simulink model "vehicle_lateral_model"  (Simulink 8.2)
settings: Solver=ode45  StartTime=0.0  StopTime=Tfinal  RelTol=1e-3
values from neighbouring files (symbols this model uses):
  Calpha = 39000    [vehicle_lateral_model_setup.m]
  Izz = 5428    [vehicle_lateral_model_setup.m]
  K = 19    [vehicle_lateral_model_setup.m]
  lf = 1.488    [vehicle_lateral_model_setup.m]
  lr = 1.712    [vehicle_lateral_model_setup.m]
  m = 2045    [vehicle_lateral_model_setup.m]
  mu = 0.9    [vehicle_lateral_model_setup.m]
  SteerAngle = 3*pi/180    (= 0.0523598775598)    [vehicle_lateral_model_setup.m]
  Vx_const = 80/3.6    (= 22.2222222222)    [vehicle_lateral_model_setup.m]
  Vy0 = 0    [vehicle_lateral_model_setup.m]
  X0 = 0    [vehicle_lateral_model_setup.m]
  Y0 = 0    [vehicle_lateral_model_setup.m]
  Yaw0 = 0    [vehicle_lateral_model_setup.m]
  yaw_rate0 = 0    [vehicle_lateral_model_setup.m]
settings Model: Creator=user  LastModifiedBy=edward
settings OptimizationCC: InitFltsAndDblsToZero=on

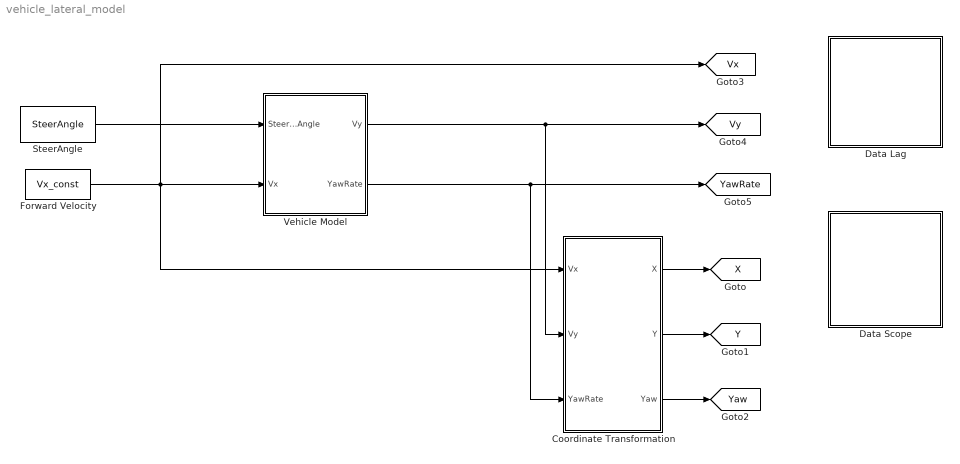
== system vehicle_lateral_model ==
  Coordinate Transformation : Subsystem
  Data Lag : Subsystem
  Data Scope : Subsystem
  Forward Velocity : Constant  Value=Vx_const
  SteerAngle : Constant  Value=SteerAngle
  Vehicle Model : Subsystem
  tag scope: Vx=global, Vy=global, X=global, Y=global, Yaw=global, YawRate=global
  wires:
  SteerAngle/1 -> Vehicle Model/1(Steering_Angle)
  Forward Velocity/1 -> Vehicle Model/2(Vx), [Vx], Coordinate Transformation/1(Vx)
  Vehicle Model/1(Vy) -> Coordinate Transformation/2(Vy), [Vy]
  Vehicle Model/2(YawRate) -> Coordinate Transformation/3(YawRate), [YawRate]
  Coordinate Transformation/1(X) -> [X]
  Coordinate Transformation/2(Y) -> [Y]
  Coordinate Transformation/3(Yaw) -> [Yaw]

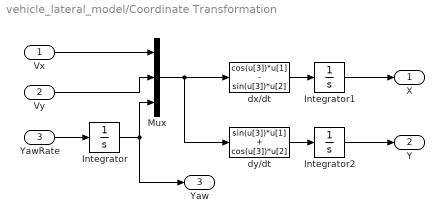
== system vehicle_lateral_model/Coordinate Transformation ==
  Vx : Inport
  Vy : Inport  Port=2
  YawRate : Inport  Port=3
  Integrator : Integrator  InitialCondition=Yaw0
  Integrator1 : Integrator  InitialCondition=X0
  Integrator2 : Integrator  InitialCondition=Y0
  Mux : Mux  Inputs=3
  dx/dt : Fcn  Expr=cos(u[3])*u[1] - sin(u[3])*u[2]
  dy/dt : Fcn  Expr=sin(u[3])*u[1] + cos(u[3])*u[2]
  X : Outport
  Y : Outport  Port=2
  Yaw : Outport  Port=3
  wires:
  YawRate/1 -> Integrator/1
  Vx/1 -> Mux/1
  Vy/1 -> Mux/2
  Integrator/1 -> Mux/3, Yaw/1
  Mux/1 -> dx/dt/1, dy/dt/1
  dx/dt/1 -> Integrator1/1
  Integrator1/1 -> X/1
  dy/dt/1 -> Integrator2/1
  Integrator2/1 -> Y/1

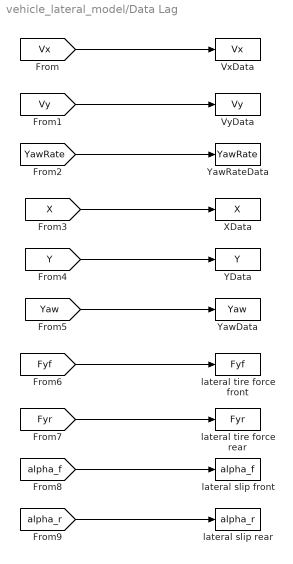
== system vehicle_lateral_model/Data Lag ==
  VxData : ToWorkspace  VariableName=Vx  SampleTime=-1
  VyData : ToWorkspace  VariableName=Vy  SampleTime=-1
  XData : ToWorkspace  VariableName=X  SampleTime=-1
  YData : ToWorkspace  VariableName=Y  SampleTime=-1
  YawData : ToWorkspace  VariableName=Yaw  SampleTime=-1
  YawRateData : ToWorkspace  VariableName=YawRate  SampleTime=-1
  lateral slip front : ToWorkspace  VariableName=alpha_f  SampleTime=-1
  lateral slip rear : ToWorkspace  VariableName=alpha_r  SampleTime=-1
  lateral tire force front : ToWorkspace  VariableName=Fyf  SampleTime=-1
  lateral tire force rear : ToWorkspace  VariableName=Fyr  SampleTime=-1
  wires:
  [Vx] -> VxData/1
  [Vy] -> VyData/1
  [YawRate] -> YawRateData/1
  [X] -> XData/1
  [Y] -> YData/1
  [Yaw] -> YawData/1
  [Fyf] -> lateral tire force front/1
  [Fyr] -> lateral tire force rear/1
  [alpha_f] -> lateral slip front/1
  [alpha_r] -> lateral slip rear/1

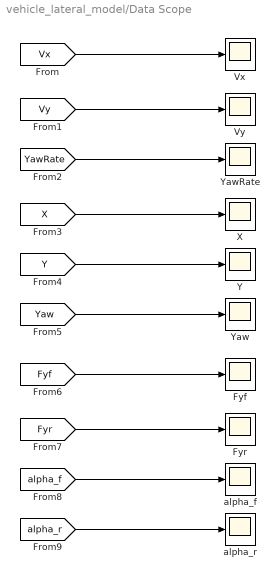
== system vehicle_lateral_model/Data Scope ==
  Fyf : Scope
  Fyr : Scope
      settings: SaveName=ScopeData3
  Vx : Scope
      settings: SaveName=ScopeData2
  Vy : Scope
      settings: SaveName=ScopeData4
  X : Scope
      settings: YMin=73.5393  YMax=81.2803  SaveName=ScopeData5
  Y : Scope
      settings: SaveName=ScopeData6
  Yaw : Scope
      settings: SaveName=ScopeData10
  YawRate : Scope
      settings: YMin=23.7489  YMax=26.2487  SaveName=ScopeData11
  alpha_f : Scope
      settings: YMin=23.7489  YMax=26.2487  SaveName=ScopeData8
  alpha_r : Scope
      settings: YMin=73.5393  YMax=81.2803  SaveName=ScopeData7
  wires:
  [Vx] -> Vx/1
  [Vy] -> Vy/1
  [YawRate] -> YawRate/1
  [X] -> X/1
  [Y] -> Y/1
  [Yaw] -> Yaw/1
  [Fyf] -> Fyf/1
  [Fyr] -> Fyr/1
  [alpha_f] -> alpha_f/1
  [alpha_r] -> alpha_r/1

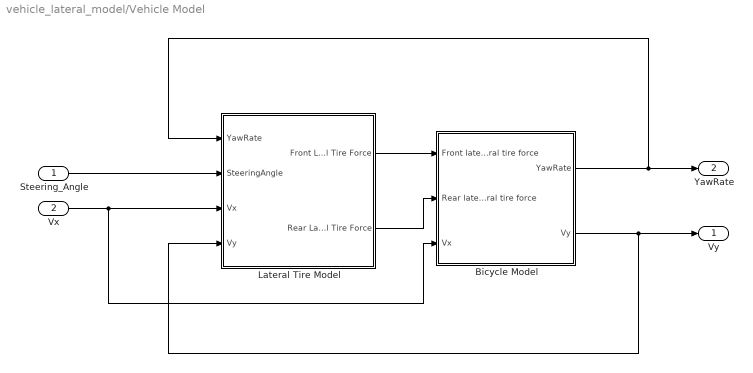
== system vehicle_lateral_model/Vehicle Model ==
  Steering_Angle : Inport
  Vx : Inport  Port=2
  Bicycle Model : Subsystem
  Lateral Tire Model : Subsystem
  Vy : Outport
  YawRate : Outport  Port=2
  wires:
  Steering_Angle/1 -> Lateral Tire Model/2(SteeringAngle)
  Lateral Tire Model/1(Front Lateral Tire Force) -> Bicycle Model/1(Front lateral tire force)
  Lateral Tire Model/2(Rear Lateral Tire Force) -> Bicycle Model/2(Rear lateral tire force)
  Bicycle Model/1(YawRate) -> Lateral Tire Model/1(YawRate), YawRate/1
  Bicycle Model/2(Vy) -> Vy/1, Lateral Tire Model/4(Vy)
  Vx/1 -> Lateral Tire Model/3(Vx), Bicycle Model/3(Vx)

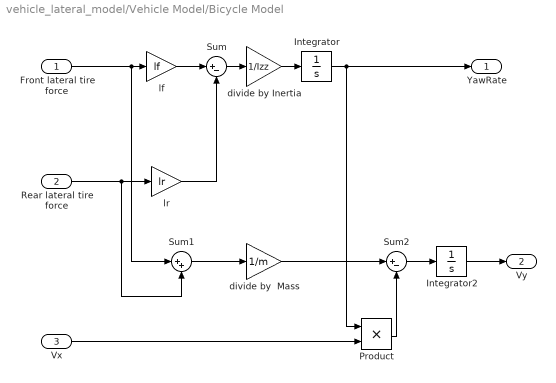
== system vehicle_lateral_model/Vehicle Model/Bicycle Model ==
  Front lateral tire force : Inport
  Rear lateral tire force : Inport  Port=2
  Vx : Inport  Port=3
  Integrator : Integrator  InitialCondition=yaw_rate0
  Integrator2 : Integrator  InitialCondition=Vy0
  Product : Product  RndMeth=Zero
  Sum : Sum  Inputs=|+-
  Sum1 : Sum  Inputs=|++
  Sum2 : Sum  Inputs=|+-
  divide by Inertia : Gain  Gain=1/Izz
  divide by  Mass : Gain  Gain=1/m
  lf : Gain  Gain=lf
  lr : Gain  Gain=lr
  YawRate : Outport
  Vy : Outport  Port=2
  wires:
  Front lateral tire force/1 -> lf/1, Sum1/1
  Rear lateral tire force/1 -> lr/1, Sum1/2
  lf/1 -> Sum/1
  lr/1 -> Sum/2
  Sum/1 -> divide by Inertia/1
  divide by Inertia/1 -> Integrator/1
  Integrator/1 -> YawRate/1, Product/1
  Sum1/1 -> divide by  Mass/1
  divide by  Mass/1 -> Sum2/1
  Vx/1 -> Product/2
  Product/1 -> Sum2/2
  Sum2/1 -> Integrator2/1
  Integrator2/1 -> Vy/1

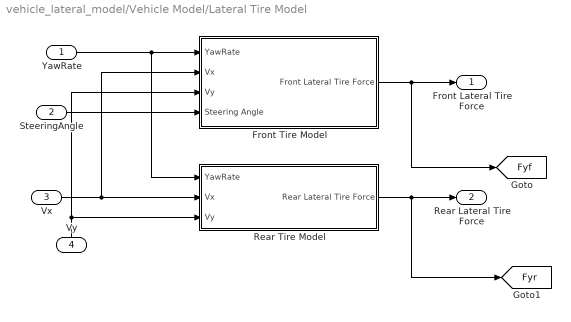
== system vehicle_lateral_model/Vehicle Model/Lateral Tire Model ==
  YawRate : Inport
  SteeringAngle : Inport  Port=2
  Vx : Inport  Port=3
  Vy : Inport  Port=4
  Front Tire Model : Subsystem
  Rear Tire Model : Subsystem
  Front Lateral Tire Force : Outport
  Rear Lateral Tire Force : Outport  Port=2
  tag scope: Fyf=global, Fyr=global
  wires:
  Vx/1 -> Rear Tire Model/2(Vx), Front Tire Model/2(Vx)
  Vy/1 -> Rear Tire Model/3(Vy), Front Tire Model/3(Vy)
  YawRate/1 -> Front Tire Model/1(YawRate), Rear Tire Model/1(YawRate)
  Front Tire Model/1(Front Lateral Tire Force) -> Front Lateral Tire Force/1, [Fyf]
  SteeringAngle/1 -> Front Tire Model/4(Steering Angle)
  Rear Tire Model/1(Rear Lateral Tire Force) -> Rear Lateral Tire Force/1, [Fyr]

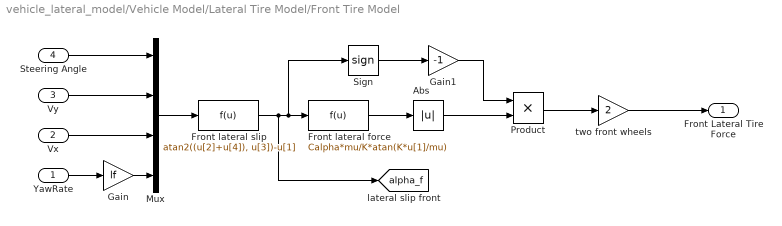
== system vehicle_lateral_model/Vehicle Model/Lateral Tire Model/Front Tire Model ==
  YawRate : Inport
  Vx : Inport  Port=2
  Vy : Inport  Port=3
  Steering Angle : Inport  Port=4
  Abs : Abs
  Front lateral force : Fcn  Expr=Calpha*mu/K*atan(K*u[1]/mu)
  Front lateral slip : Fcn  Expr=atan2((u[2]+u[4]), u[3])-u[1]
  Gain : Gain  Gain=lf
  Gain1 : Gain  Gain=-1
  Mux : Mux
  Product : Product  RndMeth=Zero
  Sign : Signum
  two front wheels : Gain  Gain=2
  Front Lateral Tire Force : Outport
  tag scope: alpha_f=global
  wires:
  Steering Angle/1 -> Mux/1
  Vy/1 -> Mux/2
  Vx/1 -> Mux/3
  YawRate/1 -> Gain/1
  Mux/1 -> Front lateral slip/1
  Gain/1 -> Mux/4
  Front lateral slip/1 -> [alpha_f], Front lateral force/1, Sign/1
  Front lateral force/1 -> Abs/1
  Sign/1 -> Gain1/1
  Gain1/1 -> Product/1
  Abs/1 -> Product/2
  Product/1 -> two front wheels/1
  two front wheels/1 -> Front Lateral Tire Force/1

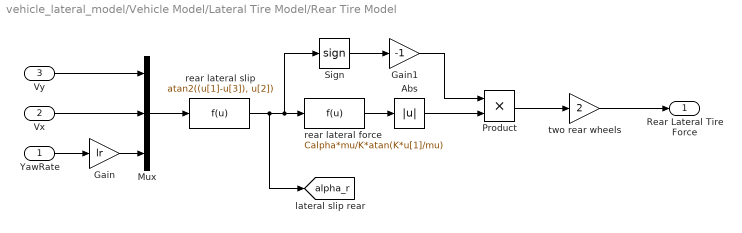
== system vehicle_lateral_model/Vehicle Model/Lateral Tire Model/Rear Tire Model ==
  YawRate : Inport
  Vx : Inport  Port=2
  Vy : Inport  Port=3
  Abs : Abs
  Gain : Gain  Gain=lr
  Gain1 : Gain  Gain=-1
  Mux : Mux  Inputs=3
  Product : Product  RndMeth=Zero
  Sign : Signum
  rear lateral force : Fcn  Expr=Calpha*mu/K*atan(K*u[1]/mu)
  rear lateral slip : Fcn  Expr=atan2((u[1]-u[3]), u[2])
  two rear wheels : Gain  Gain=2
  Rear Lateral Tire Force : Outport
  tag scope: alpha_r=global
  wires:
  rear lateral slip/1 -> [alpha_r], rear lateral force/1, Sign/1
  Gain/1 -> Mux/3
  Mux/1 -> rear lateral slip/1
  YawRate/1 -> Gain/1
  Vy/1 -> Mux/1
  Vx/1 -> Mux/2
  Sign/1 -> Gain1/1
  rear lateral force/1 -> Abs/1
  Gain1/1 -> Product/1
  Abs/1 -> Product/2
  Product/1 -> two rear wheels/1
  two rear wheels/1 -> Rear Lateral Tire Force/1
